simulink model "Tem_control_identification"  (R2025a)
settings: Solver=FixedStepDiscrete  StartTime=0.0  StopTime=600  FixedStep=1  RelTol=1e-3  EnableMultiTasking=on
libraries: arduinolib x1
settings Model: SILPILModeSetting=veronly  ExtModeTrigDuration=2  Creator=salem  LastModifiedBy=jctib
settings SolverCC: AutoInsertRateTranBlk=on
settings OptimizationCC: EnhancedBackFolding=on  PassReuseOutputArgsThreshold=0.0  MaxStackSize=64  OptimizeBlockOrder=speed  DifferentSizesBufferReuse=on  OptimizationCustomize=off
settings DebuggingCC: ParameterTunabilityLossMsg=error
settings HardwareCC: ProdBitPerPointer=32.0  ProdBitPerSizeT=32.0  ProdBitPerPtrDiffT=32.0  ProdLargestAtomicInteger=Long  ProdLargestAtomicFloat=Double  ProdWordSize=32.0  ProdHWDeviceType=ARM Compatible->ARM Cortex  UseEmbeddedCoderFeatures=off  UseSimulinkCoderFeatures=off
settings SFSimCC: MATLABDynamicMemAlloc=off
settings RTWCC: SystemTargetFile=ert.tlc  HardwareBoard=ESP32-WROOM (Arduino Compatible)  TLCOptions="-aInlineSetEventsForThisBaseRateFcn=TLC_FALSE -aSuppressMultiTaskScheduler=TLC_FALSE  -aRateBasedStepFcn=0"  TemplateMakefile=ert_default_tmf  Toolchain=ESP32  BuildConfiguration=Faster Runs  Description=Embedded Coder
settings CodeAppCC: ForceParamTrailComments=on  OperatorAnnotations=on
settings ERTTargetCC: ExtModeTransport=3.0  ExtModeAutomaticAllocSize=off  ExtModeStaticAllocSize=65536.0  InlinedParameterPlacement=Hierarchical  ERTCustomFileBanners=off  SupportContinuousTime=on  SupportNonInlinedSFcns=on  RemoveResetFunc=off  SupportVariableSizeSignals=on  ModelStepFunctionPrototypeControlCompliant=off

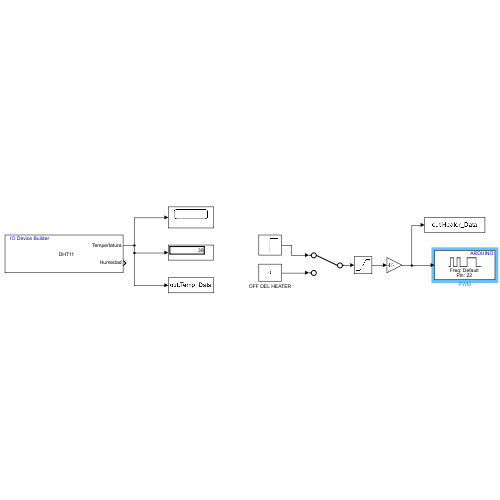
[thumbnail: Simulink's stored preview of the top-level diagram]
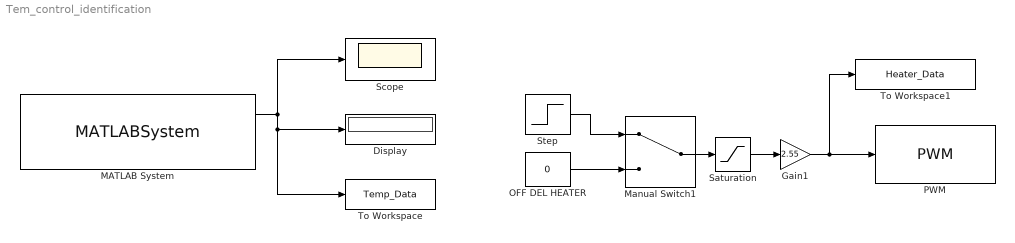
== system Tem_control_identification ==
  Display : Display
  Gain1 : Gain  Gain=2.55
  MATLAB System : MATLABSystem  System=DHT11  BlockParameter=uint32( 0 )  SampleTime=1
      mask Type: DHT11
  Manual Switch1 : ManualSwitch
  OFF DEL HEATER : Constant  Value=0
  PWM : arduinolib/PWM  pinNumber=22  frequencyType=Default  desiredFrequency=490.2  achievableFrequency=490.2
  Saturation : Saturate  UpperLimit=100  LowerLimit=0  OutDataTypeStr=Inherit: Inherit via back propagation
  Scope : Scope
      settings: ActiveDisplayYMinimum=21.701677615363643  ActiveDisplayYMaximum=59.901982912047529
  Step : Step  Time=100  After=50  SampleTime=1
  To Workspace : ToWorkspace  VariableName=Temp_Data  SampleTime=-1
      settings: Save2DSignal=2-D array (concatenate along first dimension)
  To Workspace1 : ToWorkspace  VariableName=Heater_Data  SaveFormat=Structure With Time  SampleTime=-1
      settings: Save2DSignal=2-D array (concatenate along first dimension)
  wires:
  MATLAB System/1 -> Scope/1, To Workspace/1, Display/1
  OFF DEL HEATER/1 -> Manual Switch1/2
  Saturation/1 -> Gain1/1
  Manual Switch1/1 -> Saturation/1
  Gain1/1 -> PWM/1, To Workspace1/1
  Step/1 -> Manual Switch1/1
